simulink library "epos_robot_library"  (R2022b)
settings: Solver=VariableStepAuto  StartTime=0.0  StopTime=10.0  RelTol=1e-3
libraries: simulink x4, $bdroot x1
settings Model: Creator=Nick  LastModifiedBy=Nick

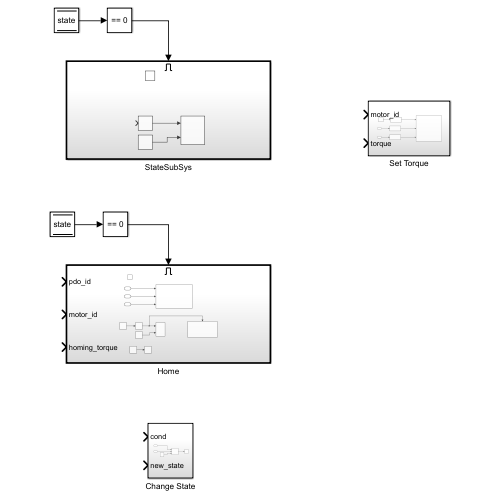
[thumbnail: Simulink's stored preview of the top-level diagram]
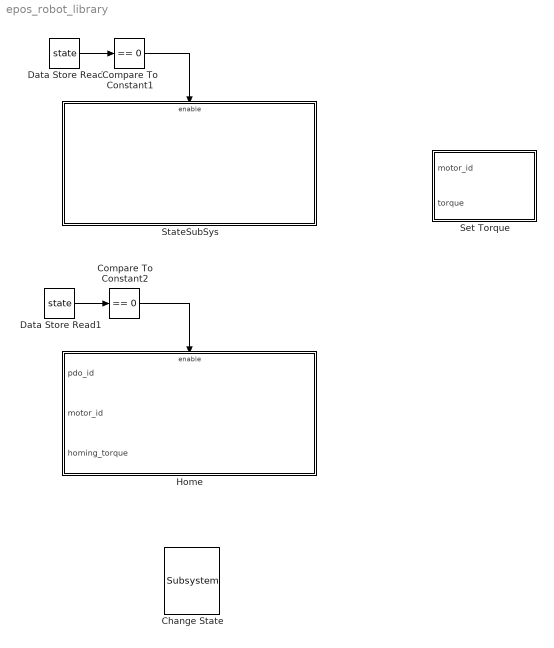
== system epos_robot_library ==
  Change State : $bdroot/Home/Subsystem  SystemSampleTime=-1  VariantActivationTime=update diagram  Latency=0  AutoFrameSizeCalculation=off
  Compare To Constant1 : simulink/Logic and Bit Operations/Compare To Constant  relop===  const=0  OutDataTypeStr=boolean
  Compare To Constant2 : simulink/Logic and Bit Operations/Compare To Constant  relop===  const=0  OutDataTypeStr=boolean
  Data Store Read : DataStoreRead  DataStoreName=state  IndexOptions=Index vector (dialog)  Indices=1  OutputSizes=1
  Data Store Read1 : DataStoreRead  DataStoreName=state  IndexOptions=Index vector (dialog)  Indices=1  OutputSizes=1
  Home : Subsystem
  Set Torque : Subsystem
  StateSubSys : Subsystem
  wires:
  Compare To Constant1/1 -> StateSubSys/Enable
  Data Store Read/1 -> Compare To Constant1/1
  Data Store Read1/1 -> Compare To Constant2/1
  Compare To Constant2/1 -> Home/Enable

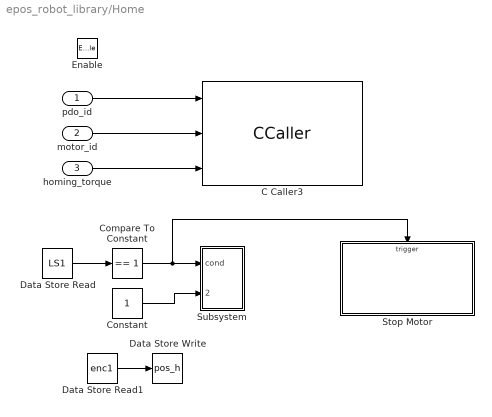
== system epos_robot_library/Home ==
  pdo_id : Inport
  motor_id : Inport  Port=2
  homing_torque : Inport  Port=3
  Enable : EnablePort
  C Caller3 : CCaller  FunctionName=set_motor  PortSpecificationStruct="%)30     .    B 4   8    (     @         %    \"     ,    !     0         %  0 \"0    $    _    07)G3F%M90  4&]R=$YA;64 4V-O<&4     26YD97@     5'EP90      4VEZ90      27-';&]B86P   X    X    !@    @    $          4    (     0    8    !         !     &    <&1O7VED   .    .     8    (    !          %    \"     $    &     0         0    !@   '!D;U]I9   #@   #@    &    \"     0         !0    @    !    !0    $         $     4   !);G!U=     X    X    !@    @    &          4    (     0    $    !          D    (               .    .     8    (    !          %    \"     $    %     0         0    !0   &EN=#,R    #@   #     &    \"     0         !0    @    !     0    $         $  ! #$    .    ,     8    (    \"0(        %    \"     $    !     0         \"  $       X    X    !@    @    $          4    (     0    @    !         !     (    ;6]T;W)?:60.    .     8    (    !          %    \"     $    (     0         0    \"    &UO=&]R7VED#@   #@    &    \"     0         !0    @    !    !0    $         $     4   !);G!U=     X    X    !@    @    &          4    (     0    $    !          D    (            \\#\\.    .     8    (    !          %    \"     $    %     0         0    !0   &EN=#,R    #@   #     &    \"     0         !0    @    !     0    $         $  ! #$    .    ,     8    (    \"0(        %    \"     $    !     0         \"  $       X    X    !@    @    $          4    (     0    <    !         !     '    <V5T7W9A;  .    .     8    (    !          %    \"     $    '     0         0    !P   '-E=%]V86P #@   #@    &    \"     0         !0    @    !    !0    $         $     4   !);G!U=     X    X    !@    @    &          4    (     0    $    !          D    (             $ .    .     8    (    !          %    \"     $    &     0         0    !@   &1O=6)L90  #@   #     &    \"     0         !0    @    !     0    $         $  ! #$    .    ,     8    (    \"0(        %    \"     $    !     0         \"  $"  SampleTime=0.01
  Compare To Constant : simulink/Logic and Bit Operations/Compare To Constant  relop===  const=1  OutDataTypeStr=boolean
  Constant : Constant
  Data Store Read : DataStoreRead  DataStoreName=LS1  IndexOptions=Index vector (dialog)  Indices=1  OutputSizes=1
  Data Store Read1 : DataStoreRead  DataStoreName=enc1  IndexOptions=Index vector (dialog)  Indices=1  OutputSizes=1
  Data Store Write : DataStoreWrite  DataStoreName=pos_h  IndexOptions=Index vector (dialog)  Indices=1  OutputSizes=1
  Stop Motor : Subsystem  TreatAsAtomicUnit=on
  Subsystem : Subsystem
  wires:
  Compare To Constant/1 -> Stop Motor/Trigger, Subsystem/1(cond)
  motor_id/1 -> C Caller3/2
  pdo_id/1 -> C Caller3/1
  homing_torque/1 -> C Caller3/3
  Data Store Read/1 -> Compare To Constant/1
  Constant/1 -> Subsystem/2(new_state)
  Data Store Read1/1 -> Data Store Write/1

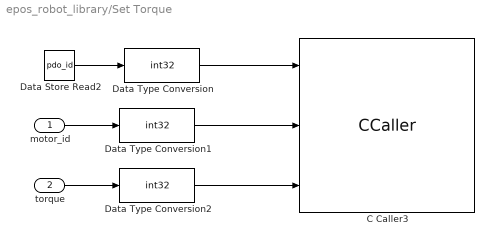
== system epos_robot_library/Set Torque ==
  motor_id : Inport
  torque : Inport  Port=2
  C Caller3 : CCaller  FunctionName=set_motor  PortSpecificationStruct="%)30     .    B 4   8    (     @         %    \"     ,    !     0         %  0 \"0    $    _    07)G3F%M90  4&]R=$YA;64 4V-O<&4     26YD97@     5'EP90      4VEZ90      27-';&]B86P   X    X    !@    @    $          4    (     0    8    !         !     &    <&1O7VED   .    .     8    (    !          %    \"     $    &     0         0    !@   '!D;U]I9   #@   #@    &    \"     0         !0    @    !    !0    $         $     4   !);G!U=     X    X    !@    @    &          4    (     0    $    !          D    (               .    .     8    (    !          %    \"     $    %     0         0    !0   &EN=#,R    #@   #     &    \"     0         !0    @    !     0    $         $  ! #$    .    ,     8    (    \"0(        %    \"     $    !     0         \"  $       X    X    !@    @    $          4    (     0    @    !         !     (    ;6]T;W)?:60.    .     8    (    !          %    \"     $    (     0         0    \"    &UO=&]R7VED#@   #@    &    \"     0         !0    @    !    !0    $         $     4   !);G!U=     X    X    !@    @    &          4    (     0    $    !          D    (            \\#\\.    .     8    (    !          %    \"     $    %     0         0    !0   &EN=#,R    #@   #     &    \"     0         !0    @    !     0    $         $  ! #$    .    ,     8    (    \"0(        %    \"     $    !     0         \"  $       X    X    !@    @    $          4    (     0    <    !         !     '    <V5T7W9A;  .    .     8    (    !          %    \"     $    '     0         0    !P   '-E=%]V86P #@   #@    &    \"     0         !0    @    !    !0    $         $     4   !);G!U=     X    X    !@    @    &          4    (     0    $    !          D    (             $ .    .     8    (    !          %    \"     $    &     0         0    !@   &1O=6)L90  #@   #     &    \"     0         !0    @    !     0    $         $  ! #$    .    ,     8    (    \"0(        %    \"     $    !     0         \"  $"
  Data Store Read2 : DataStoreRead  DataStoreName=pdo_id  IndexOptions=Index vector (dialog)  Indices=1  OutputSizes=1
  Data Type Conversion : DataTypeConversion  OutDataTypeStr=int32  SaturateOnIntegerOverflow=off  RndMeth=Floor
  Data Type Conversion1 : DataTypeConversion  OutDataTypeStr=int32  SaturateOnIntegerOverflow=off  RndMeth=Floor
  Data Type Conversion2 : DataTypeConversion  OutDataTypeStr=int32  SaturateOnIntegerOverflow=off  RndMeth=Floor
  wires:
  motor_id/1 -> Data Type Conversion1/1
  torque/1 -> Data Type Conversion2/1
  Data Store Read2/1 -> Data Type Conversion/1
  Data Type Conversion/1 -> C Caller3/1
  Data Type Conversion1/1 -> C Caller3/2
  Data Type Conversion2/1 -> C Caller3/3

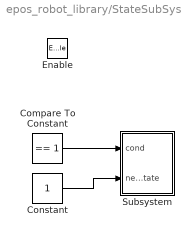
== system epos_robot_library/StateSubSys ==
  Enable : EnablePort
  Compare To Constant : simulink/Logic and Bit Operations/Compare To Constant  relop===  const=1  OutDataTypeStr=boolean
  Constant : Constant
  Subsystem : Subsystem
  wires:
  Compare To Constant/1 -> Subsystem/1(cond)
  Constant/1 -> Subsystem/2(new_state)

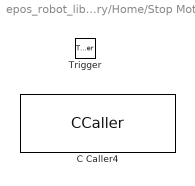
== system epos_robot_library/Home/Stop Motor ==
  Trigger : TriggerPort  VariantControl=(inherit)
  C Caller4 : CCaller  FunctionName=stop_motor  SampleTime=0.001

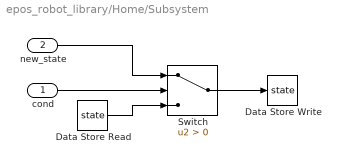
== system epos_robot_library/Home/Subsystem ==
  cond : Inport
  new_state : Inport  Port=2
  Data Store Read : DataStoreRead  DataStoreName=state  IndexOptions=Index vector (dialog)  Indices=1  OutputSizes=1
  Data Store Write : DataStoreWrite  DataStoreName=state  IndexOptions=Index vector (dialog)  Indices=1  OutputSizes=1
  Switch : Switch  Criteria=u2 > Threshold  SaturateOnIntegerOverflow=off  InputSameDT=off
  wires:
  new_state/1 -> Switch/1
  Data Store Read/1 -> Switch/3
  Switch/1 -> Data Store Write/1
  cond/1 -> Switch/2

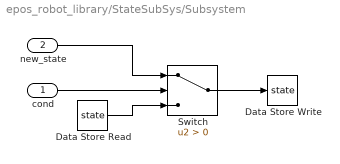
== system epos_robot_library/StateSubSys/Subsystem ==
  cond : Inport
  new_state : Inport  Port=2
  Data Store Read : DataStoreRead  DataStoreName=state  IndexOptions=Index vector (dialog)  Indices=1  OutputSizes=1
  Data Store Write : DataStoreWrite  DataStoreName=state  IndexOptions=Index vector (dialog)  Indices=1  OutputSizes=1
  Switch : Switch  Criteria=u2 > Threshold  SaturateOnIntegerOverflow=off  InputSameDT=off
  wires:
  new_state/1 -> Switch/1
  Data Store Read/1 -> Switch/3
  Switch/1 -> Data Store Write/1
  cond/1 -> Switch/2
